simulink model "wlan80211BeaconRx"  (R2015b)
settings: Solver=FixedStepDiscrete  SolverMode=SingleTasking  StartTime=0.0  StopTime=inf  RelTol=1e-3
PreLoadFcn:
  | sample = 860*2816;
  | load('commwlan80211BusTypes')
  | openMPDUGUI = true;
PostLoadFcn:
  | commwlan80211BeaconRxModelParams('init')
  | commwlan80211BeaconRxModelParams('scope')
InitFcn:
  | load('commwlan80211BusTypes')
  | commwlan80211BeaconRxModelParams('init')
model workspace: external: MAT-File (data not in the file)
undefined symbols (not defined in the file or in its folder): p80211
libraries: commwlan80211BeaconLib x6, commdigbbndpm3 x1, commsequence2 x1, commrfcorlib x1, commfilt2 x1, simulink x1
CloseFcn:
  | hFig = findall(0, 'Type', 'figure', 'Name', '802.11 Beacon Frame');
  | if ishghandle(hFig)
  | close(hFig);
  | end
  | clear hFig
  | if (exist('ans')==1) && (iscell(ans) && (numel(ans) == 0))
  | clear ans
  | end
Description:
  | IEEE 802.11 WLAN Beacon Frame Receiver for Captured Data
  | 
  | This example shows how to process a captured beacon frame and display the
  | frame information.
settings Model: Creator=The MathWorks, Inc.  LastModifiedBy=DPu1
settings DataIOCC: SaveFormat=Array  SaveOutput=off  SignalLogging=off  DSMLogging=off  SaveTime=off
settings OptimizationCC: DefaultParameterBehavior=Inlined  InlineInvariantSignals=on  ExpressionDepthLimit=2147483647  EfficientFloat2IntCast=on
settings DebuggingCC: UnderspecifiedInitializationDetection=Classic  MergeDetectMultiDrivingBlocksExec=none  SolverPrmCheckMsg=warning  UniqueDataStoreMsg=error  StateNameClashWarn=warning
settings HardwareCC: ProdBitPerPointer=32  ProdLargestAtomicFloat=None  ProdIntDivRoundTo=Undefined  ProdEndianess=Unspecified  ProdWordSize=32  ProdHWDeviceType=32-bit Generic
settings GRTTargetCC: GeneratePreprocessorConditionals=Disable all  CombineOutputUpdateFcns=off  GRTInterface=on
settings ConfigComp: CovModelRefEnable=Off  CovSFcnEnable=off

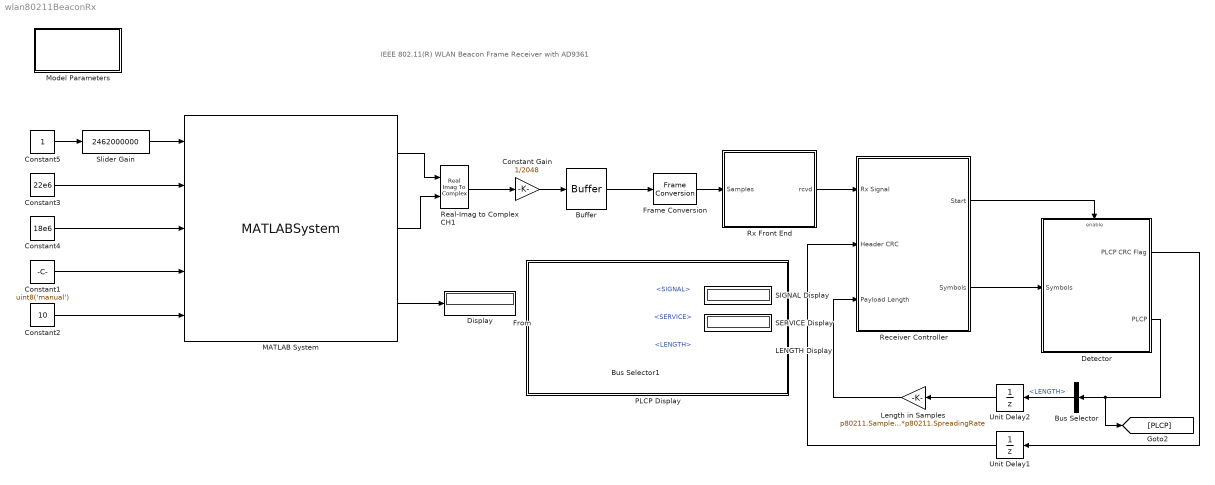
== system wlan80211BeaconRx ==
  note: IEEE 802.11(R) WLAN
      | Beacon Frame Receiver with AD9361
  Buffer : Buffer  N=2816  TreatMby1Signals=One channel
  Bus Selector : BusSelector  OutputSignals=LENGTH
  Bus Selector1 : BusSelector  OutputSignals=SIGNAL,SERVICE,LENGTH
  Constant Gain : Gain  Gain=1/2048  SaturateOnIntegerOverflow=on  ParamDataTypeStr=Inherit: Same as input
  Constant1 : Constant  Value=uint8('manual')  SampleTime=1
  Constant2 : Constant  Value=10  SampleTime=1
  Constant3 : Constant  Value=22e6  SampleTime=1
  Constant4 : Constant  Value=18e6  SampleTime=1
  Constant5 : Constant  SampleTime=1
  Detector : Subsystem
      settings: CloseFcn=clear BeaconFrameBodyType rcvd
  Display : Display
  Frame Conversion : FrameConversion  InheritSamplingMode=off
  LENGTH Display : Display
  Length in Samples : Gain  Gain=p80211.SamplesPerChip*p80211.SpreadingRate  OutDataTypeStr=uint32  SaturateOnIntegerOverflow=on  ParamDataTypeStr=Inherit: Same as input
  MATLAB System : MATLABSystem  System=iio_sys_obj  ip_address=10.66.100.86  dev_name=ad9361  in_ch_no=0  in_ch_size=sample  out_ch_no=2  out_ch_size=sample  SimulateUsing=Interpreted execution
      mask Type: iio_sys_obj
      mask Display:
      | disp('ad9361');
      | port_label('input',1,'RX_LO_FREQ');
      | port_label('input',2,'RX_SAMPLING_FREQ');
      | port_label('input',3,'RX_RF_BANDWIDTH');
      | port_label('input',4,'RX1_GAIN_MODE');
      | port_label('input',5,'RX1_GAIN');
      | port_label('output',1,'DATA_OUT1');
      | port_label('output',2,'DATA_OUT2');
      | port_label('output',3,'RX1_RSSI');
  Model Parameters : Subsystem  mask(Model Parameters){rcvdSignal=Channel 5 set 1, agcStepSize=6, agcMaxGain=60, corrThreshold=2000, sampsPerChip=2}
      mask prompts: rcvdSignal "Received signal:"; agcStepSize "AGC loop gain:"; agcMaxGain "Maximum AGC power gain in dB:"; corrThreshold "Synchronization threshold:"; sampsPerChip "Samples per chip:"
      mask help:
      | Choose 802.11 receiver parameters.
      |
      | You can select from four different saved received signals that contain 802.11 packets captured using a radio.
      |
      | You can set the AGC parameters and samples per chip used in the receiver. You can also set the synchronization threshold value to determine the correlation threshold used to declare the presence of an 802.11 packet.
      mask init:
      | commwlan80211BeaconRxModelParams('init');
      mask Help: helpview(commdhelp);
      mask TypeOptions rcvdSignal: Channel 5 set 1 | Channel 5 set 2 | Channel 9 set 1 | Channel 9 set 2
      mask TypeOptions sampsPerChip: 4 | 2
      mask Display: disp('Model\nParameters')
  PLCP Display : Subsystem
      mask Display: disp('')
  Real-Imag to Complex CH1 : RealImagToComplex  SampleTime=sample/(25e6)
  Receiver Controller : Subsystem
  Rx Front End : Subsystem
  SERVICE Display : Display
      settings: Format=hex (Stored Integer)
  SIGNAL Display : Display
      settings: Format=hex (Stored Integer)
  Slider Gain : simulink/Math Operations/Slider Gain  low=200000  gain=2462000000  high=6000000000
  Unit Delay1 : UnitDelay  InitialCondition=1  SampleTime=-1
  Unit Delay2 : UnitDelay  InitialCondition=1  SampleTime=-1
  wires:
  Length in Samples/1 -> Receiver Controller/3(Payload Length)
  Detector/1(PLCP CRC Flag) -> Unit Delay1/1
  Unit Delay1/1 -> Receiver Controller/2(Header CRC)
  Bus Selector/1 -> Unit Delay2/1  "<LENGTH>"
  Receiver Controller/1(Start) -> Detector/Enable
  Rx Front End/1(rcvd) -> Receiver Controller/1(Rx Signal)
  Unit Delay2/1 -> Length in Samples/1
  Detector/2(PLCP) -> [PLCP], Bus Selector/1
  [PLCP] -> Bus Selector1/1
  Bus Selector1/3 -> LENGTH Display/1  "<LENGTH>"
  Bus Selector1/1 -> SIGNAL Display/1  "<SIGNAL>"
  Bus Selector1/2 -> SERVICE Display/1  "<SERVICE>"
  Receiver Controller/2(Symbols) -> Detector/1(Symbols)
  Frame Conversion/1 -> Rx Front End/1(Samples)
  Real-Imag to Complex CH1/1 -> Constant Gain/1
  Constant Gain/1 -> Buffer/1
  Constant5/1 -> Slider Gain/1
  Slider Gain/1 -> MATLAB System/1
  Constant3/1 -> MATLAB System/2
  Constant4/1 -> MATLAB System/3
  Constant1/1 -> MATLAB System/4
  Constant2/1 -> MATLAB System/5
  MATLAB System/1 -> Real-Imag to Complex CH1/1
  MATLAB System/2 -> Real-Imag to Complex CH1/2
  MATLAB System/3 -> Display/1
  Buffer/1 -> Frame Conversion/1

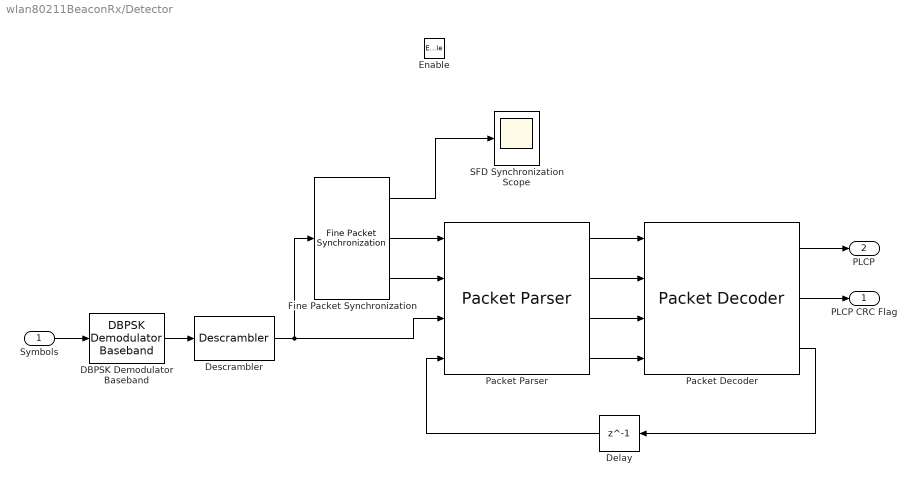
== system wlan80211BeaconRx/Detector ==
  Symbols : Inport
  Enable : EnablePort  StatesWhenEnabling=reset  PropagateVarSize=During execution
  DBPSK Demodulator Baseband : commdigbbndpm3/DBPSK Demodulator Baseband  Ph=0  outDtype=Smallest unsigned integer
  Delay : Delay  DelayLength=1  InitialCondition=0  InputProcessing=Columns as channels (frame based)
  Descrambler : commsequence2/Descrambler  M=2  poly=p80211.ScramblerPolynomial  iniStaSource=Dialog Parameter  ini_sta=[0 0 0 0 0 0 0]  resetViaPort=off
  Fine Packet Synchronization : commwlan80211BeaconLib/Fine Packet Synchronization
  Packet Decoder : commwlan80211BeaconLib/Packet Decoder
  Packet Parser : commwlan80211BeaconLib/Packet Parser
  SFD Synchronization Scope : Scope
      settings: Priority=10
  PLCP CRC Flag : Outport  InitialOutput=1
  PLCP : Outport  Port=2
  wires:
  Packet Decoder/3 -> Delay/1
  Packet Decoder/2 -> PLCP CRC Flag/1
  Packet Decoder/1 -> PLCP/1
  Packet Parser/4 -> Packet Decoder/4
  Packet Parser/3 -> Packet Decoder/3
  Packet Parser/2 -> Packet Decoder/2
  Packet Parser/1 -> Packet Decoder/1
  Delay/1 -> Packet Parser/4
  Fine Packet Synchronization/3 -> Packet Parser/2
  Fine Packet Synchronization/2 -> Packet Parser/1
  Descrambler/1 -> Packet Parser/3, Fine Packet Synchronization/1
  Symbols/1 -> DBPSK Demodulator Baseband/1
  DBPSK Demodulator Baseband/1 -> Descrambler/1
  Fine Packet Synchronization/1 -> SFD Synchronization Scope/1

== system wlan80211BeaconRx/Model Parameters ==

== system wlan80211BeaconRx/PLCP Display ==

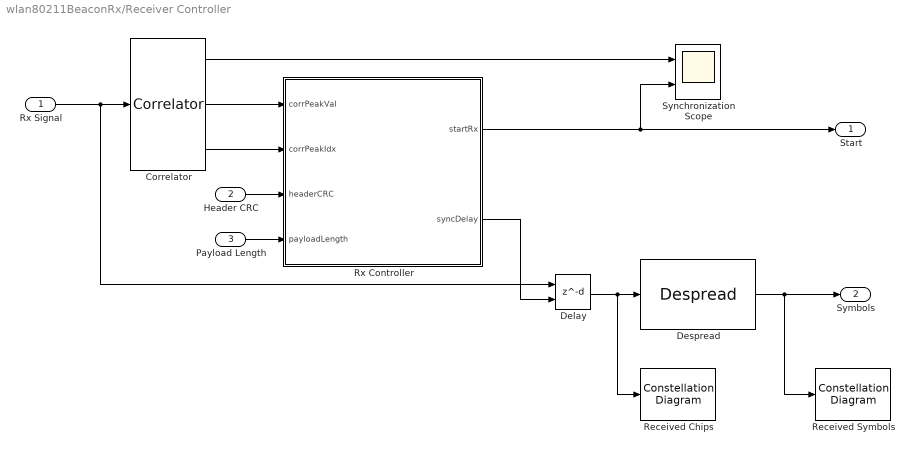
== system wlan80211BeaconRx/Receiver Controller ==
  Rx Signal : Inport
  Header CRC : Inport  Port=2
  Payload Length : Inport  Port=3
  Correlator : commwlan80211BeaconLib/Correlator
  Delay : Delay  DelayLengthSource=Input port  DelayLengthUpperLimit=p80211.SamplesPerChannelFrame  InputProcessing=Columns as channels (frame based)
      settings: InputPortMap=u0,p1
  Despread : commwlan80211BeaconLib/Despread
  Received Chips : ConstellationDiagram  Tag=ScatterPlot  Priority=1
  Received Symbols : ConstellationDiagram  Tag=ScatterPlot  Priority=2
  Rx Controller : MATLAB Function  TreatAsAtomicUnit=on
  Synchronization Scope : Scope  NumInputPorts=2
      settings: Priority=1
  Start : Outport
  Symbols : Outport  Port=2
  wires:
  Despread/1 -> Received Symbols/1, Symbols/1
  Rx Controller/2(syncDelay) -> Delay/2
  Rx Controller/1(startRx) -> Synchronization Scope/2, Start/1
  Header CRC/1 -> Rx Controller/3(headerCRC)
  Correlator/2 -> Rx Controller/1(corrPeakVal)
  Correlator/3 -> Rx Controller/2(corrPeakIdx)
  Rx Signal/1 -> Correlator/1, Delay/1
  Payload Length/1 -> Rx Controller/4(payloadLength)
  Delay/1 -> Despread/1, Received Chips/1
  Correlator/1 -> Synchronization Scope/1

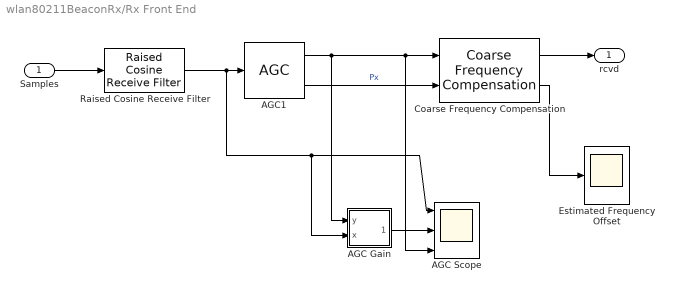
== system wlan80211BeaconRx/Rx Front End ==
  Samples : Inport
  AGC Gain : Subsystem
  AGC Scope : Scope  NumInputPorts=3
  AGC1 : commrfcorlib/AGC  LegacyMode=off  DetectorMethod=Rectifier  LoopMethod=Linear  UpdatePeriod=100  StepSize=0.1  AdaptationStepSize=p80211.AGCStepSize  DesiredOutputPower=1  AveragingLength=50  MaximumGain=30  MaxPowerGain=p80211.AGCUpperLimit  GainOutputPort=off  InputPowerOutputPort=on  SimulateUsing=Code generation
  Coarse Frequency Compensation : commwlan80211BeaconLib/Coarse Frequency Compensation  decimRate=44*p80211.SamplesPerChip/2  maxOffset=50000  M=2
  Estimated Frequency Offset : Scope
  Raised Cosine Receive Filter : commfilt2/Raised Cosine Receive Filter  filtType=Square root  N=p80211.SamplesPerChip  filtSpan=p80211.FilterOrder  currentFiltSpan=2*(p80211.FilterOrder/2)  D=p80211.FilterOrder/2  R=0.3  sampMode=Mute  saveAsFlag=0  rateMode=Downsampling  downFactor=1  downOffset=0  framing=Enforce single-rate processing  InputProcessing=Columns as channels (frame based)  checkGain=Normalized  filterGain=1  checkCoeff=off  variableName=rcRxFilt  launchFVT=off  roundingMode=Floor  overflowMode=off
  rcvd : Outport
  wires:
  Coarse Frequency Compensation/1 -> rcvd/1
  Samples/1 -> Raised Cosine Receive Filter/1
  Coarse Frequency Compensation/2 -> Estimated Frequency Offset/1
  Raised Cosine Receive Filter/1 -> AGC1/1, AGC Gain/2(x), AGC Scope/1
  AGC1/1 -> AGC Gain/1(y), Coarse Frequency Compensation/1, AGC Scope/3
  AGC1/2 -> Coarse Frequency Compensation/2  "Px"
  AGC Gain/1(gain) -> AGC Scope/2

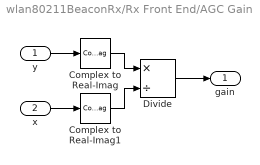
== system wlan80211BeaconRx/Rx Front End/AGC Gain ==
  y : Inport
  x : Inport  Port=2
  Complex to Real-Imag : ComplexToRealImag  Output=Real
  Complex to Real-Imag1 : ComplexToRealImag  Output=Real
  Divide : Product  Inputs=*/
  gain : Outport
  wires:
  Complex to Real-Imag/1 -> Divide/1
  x/1 -> Complex to Real-Imag1/1
  y/1 -> Complex to Real-Imag/1
  Complex to Real-Imag1/1 -> Divide/2
  Divide/1 -> gain/1

== matlab function wlan80211BeaconRx/Receiver Controller/Rx Controller ==
  data: corrPeakVal input; startRx output; corrPeakIdx input; headerCRC input boolean size=[1 1]; payloadLength input size=1; p80211 parameter; syncDelay output
function [startRx, syncDelay] = ...
  rxCtrl(corrPeakVal, corrPeakIdx, headerCRC, payloadLength, p80211)
%#codegen

persistent rxOn controllerState payloadCount lastSyncDelay corrPeakValOld

% State Enums
SearchPLCP = 0;
GetPLCP    = 2;
GetPayload = 4;

if isempty(rxOn)
  % Initialize receiver controller
  rxOn = false;
  controllerState = SearchPLCP;
  payloadCount = 0;
  lastSyncDelay = 0;
  corrPeakValOld = 0;
end

if (corrPeakValOld < corrPeakVal)
  controllerState = SearchPLCP;
end

switch controllerState
  case SearchPLCP
    % Search for the PLCP SYNC signal
    
    if corrPeakVal > p80211.CorrelationThreshold
      corrPeakValOld = corrPeakVal;
      % Synchronize to the end of the SYNC. Get 8 (scrambler length) extra
      % bits to initialize DPSK demodulator and scrambler
      scramblerLen = length(p80211.ScramblerPolynomial);
      lastSyncDelay = p80211.SamplesPerChannelFrame - (corrPeakIdx ...
        - scramblerLen*p80211.SpreadingRate*p80211.SamplesPerChip); 
      payloadCount = p80211.NumSYNCSamples ...
        - scramblerLen*p80211.SpreadingRate*p80211.SamplesPerChip;
      rxOn = true;
      
      controllerState = GetPLCP;
    end
  case GetPLCP
    % In this state we receive both SFD, which is part of PLCP preamble,
    % and the PLCP header
    
    payloadCount = payloadCount + p80211.SamplesPerChannelFrame;
    
    if (payloadCount >= ...
        (p80211.NumPLCPSamples+p80211.ScramblerAmbiguitySamples))
    % Wait one more channel frame to let the PLCP CRC result to reach.
    % There is a delay between detector and receiver controller to break
    % the algebraic loop.
      if headerCRC ~= 1
        controllerState = GetPayload;
      else
        rxOn = false;
        lastSyncDelay = 0;
        payloadCount = 0;
        controllerState = SearchPLCP;
      end
    end
  case GetPayload
    % Receive payload symbols
    
    payloadCount = payloadCount + p80211.SamplesPerChannelFrame;
    
    if payloadCount >= ...
        ((p80211.NumPLCPSamples+p80211.ScramblerAmbiguitySamples) + ...
        payloadLength)
      rxOn = false;
      lastSyncDelay = 0;
      payloadCount = 0;
      controllerState = SearchPLCP;
    end
end

startRx = rxOn;
syncDelay = lastSyncDelay;
